simulink model "los_test"  (Simulink 7.1)
settings: Solver=ode4  StartTime=0.0  StopTime=700  FixedStep=0.1  RelTol=1e-3
libraries: fordypningsprosjekt x4, simulink x1
settings Model: Creator=anderga  LastModifiedBy=anders

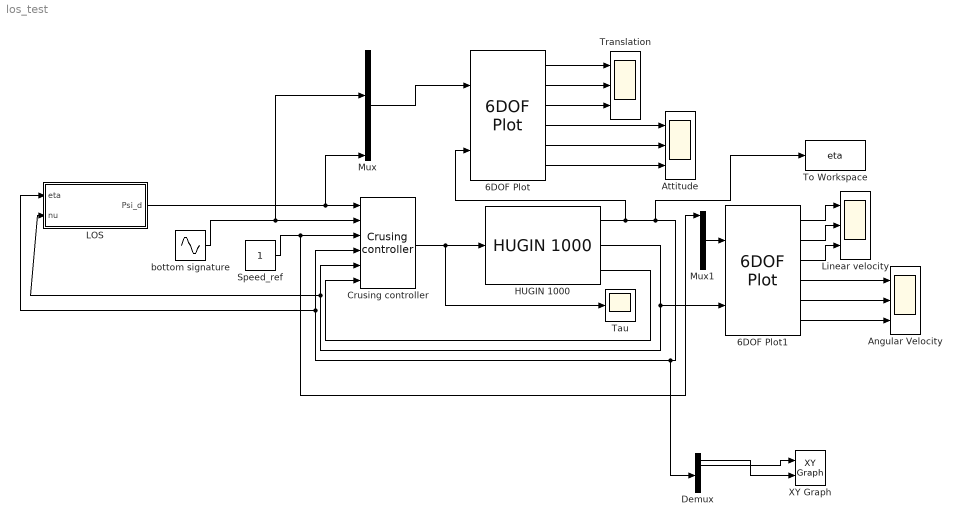
== system los_test ==
  6DOF Plot : fordypningsprosjekt/6DOF Plot  SystemSampleTime=-1
  6DOF Plot1 : fordypningsprosjekt/6DOF Plot  SystemSampleTime=-1
  Angular Velocity : Scope  NumInputPorts=3
      settings: YMin=-0.25~-0.015~-15  YMax=0.3~0.01~5  SaveName=ScopeData3
  Attitude : Scope  NumInputPorts=3
      settings: YMin=-1~-1.25~-100  YMax=0.75~0.25~200  SaveName=Attitude_ref
  Crusing controller : fordypningsprosjekt/Crusing controller  SystemSampleTime=-1  Kp_u=10  Ki_u=3  Kp_c=200  Kd_c=100  Kp_d=10  Kp2_d=10  Kd_d=5
  Demux : Demux  Outputs=6
  HUGIN 1000 : fordypningsprosjekt/HUGIN 1000  SystemSampleTime=-1  eta_0=eta0  nu_0=[0 0 0 0 0 0]  c_on_off=on  beta_c=-60  V_c=0.6
  LOS : Subsystem
  Linear velocity : Scope  NumInputPorts=3
      settings: YMin=0.75~-0.075~-0.05  YMax=1.1~0.1~0.03  SaveName=Lin_veloc
  Mux : Mux  Inputs=6
  Mux1 : Mux  Inputs=6
  Speed_ref : Constant  OutDataType=sfix(16)  OutScaling=2^0
  Tau : Scope
      settings: YMin=-55  YMax=30  SaveName=ScopeData4
  To Workspace : ToWorkspace  VariableName=eta  SampleTime=-1  SaveFormat=Structure With Time
  Translation : Scope  NumInputPorts=3
      settings: YMin=0~0~52.5  YMax=200~22.5~56  SaveName=Translation_ref
  XY Graph : simulink/Sinks/XY Graph  SystemSampleTime=-1  xmin=-1000  xmax=1000  ymin=-1000  ymax=1000  st=-1
  bottom signature : Sin  Amplitude=6  Bias=50  Frequency=0.01  SampleTime=0
  wires:
  Crusing controller/1 -> HUGIN 1000/1, Tau/1
  HUGIN 1000/1 -> 6DOF Plot/2, Crusing controller/4, LOS/1(eta), Demux/1, To Workspace/1
  HUGIN 1000/2 -> Crusing controller/5, LOS/2(nu), 6DOF Plot1/2
  HUGIN 1000/3 -> Crusing controller/6
  bottom signature/1 -> Crusing controller/2, Mux/3
  Speed_ref/1 -> Crusing controller/3, Mux1/1
  LOS/1(Psi_d) -> Crusing controller/1, Mux/6
  Mux/1 -> 6DOF Plot/1
  6DOF Plot/1 -> Translation/1
  6DOF Plot/2 -> Translation/2
  6DOF Plot/3 -> Translation/3
  6DOF Plot/4 -> Attitude/1
  6DOF Plot/5 -> Attitude/2
  6DOF Plot/6 -> Attitude/3
  Mux1/1 -> 6DOF Plot1/1
  6DOF Plot1/1 -> Linear velocity/1
  6DOF Plot1/2 -> Linear velocity/2
  6DOF Plot1/3 -> Linear velocity/3
  6DOF Plot1/4 -> Angular Velocity/1
  6DOF Plot1/5 -> Angular Velocity/2
  6DOF Plot1/6 -> Angular Velocity/3
  Demux/1 -> XY Graph/2
  Demux/2 -> XY Graph/1

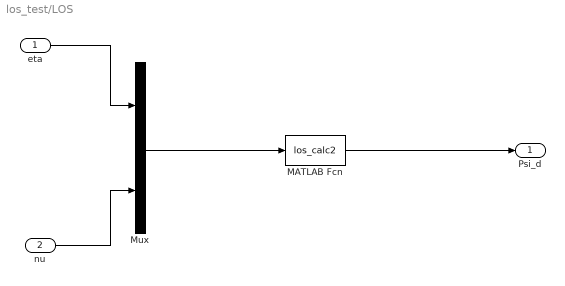
== system los_test/LOS ==
  eta : Inport  OutDataType=sfix(16)  OutScaling=2^0
  nu : Inport  Port=2  OutDataType=sfix(16)  OutScaling=2^0
  MATLAB Fcn : MATLABFcn  MATLABFcn=los_calc2  OutputDimensions=1
  Mux : Mux  Inputs=2
  Psi_d : Outport  OutDataType=sfix(16)  OutScaling=2^0
  wires:
  eta/1 -> Mux/1
  nu/1 -> Mux/2
  Mux/1 -> MATLAB Fcn/1
  MATLAB Fcn/1 -> Psi_d/1
